simulink model "Aufgabe_5_Simu"  (Simulink 9.2)
settings: Solver=ode45  StartTime=0  StopTime=100  RelTol=1e-3  EnableMultiTasking=on
InitFcn:
  | Ts = 0.1;  % Nicht entfernen!!!
settings Model: Creator=ST  LastModifiedBy=danial
settings SolverCC: ZeroCrossAlgorithm=Adaptive
settings DataIOCC: SignalLoggingSaveFormat=Dataset
settings DebuggingCC: IgnoredZcDiagnostic=none  SolverPrmCheckMsg=warning  FcnCallInpInsideContextMsg=error
settings GRTTargetCC: CombineOutputUpdateFcns=on  GRTInterface=off
settings ConfigComp: CovSFcnEnable=off

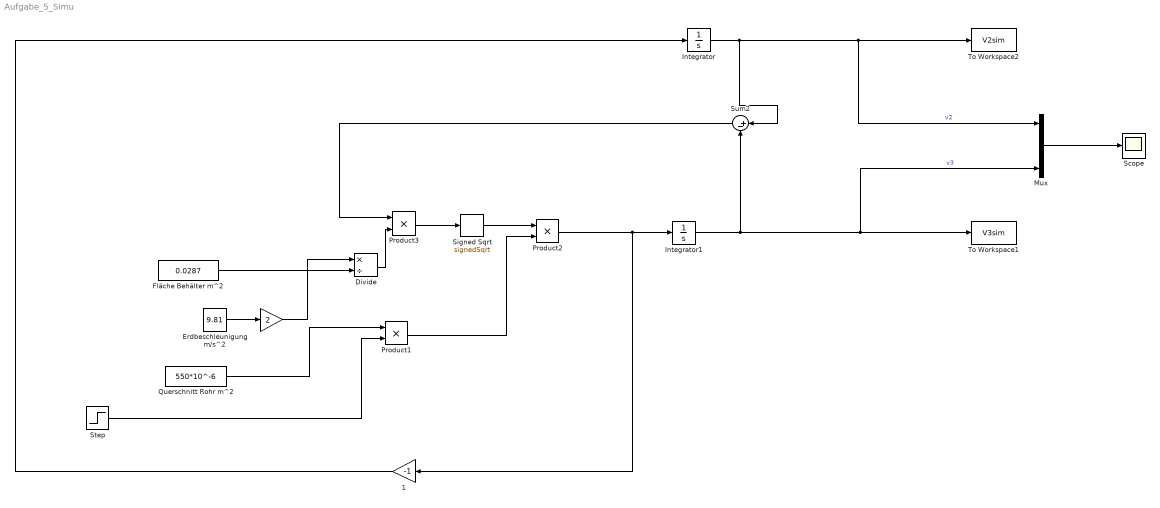
== system Aufgabe_5_Simu ==
  " " : Gain  Gain=2
  " 1" : Gain  Gain=-1
  Divide : Product  Inputs=*/
  Erdbeschleunigung m/s^2 : Constant  Value=9.81  OutDataTypeStr=double
  Fläche Behälter m^2 : Constant  Value=0.0287  OutDataTypeStr=double
  Integrator : Integrator  InitialCondition=9.2*10^-3  LimitOutput=on  UpperSaturationLimit=10*10^-3
  Integrator1 : Integrator  InitialCondition=2.6*10^-3  LimitOutput=on  UpperSaturationLimit=10*10^-3
  Mux : Mux  Inputs=3
  Product1 : Product
  Product2 : Product
  Product3 : Product
  Querschnitt Rohr m^2 : Constant  Value=550*10^-6  OutDataTypeStr=double
  Scope : Scope
  Signed Sqrt : Sqrt  Operator=signedSqrt  SaturateOnIntegerOverflow=on
  Step : Step  Time=2  SampleTime=0
  Sum2 : Sum  Inputs=|+-
  To Workspace1 : ToWorkspace  VariableName=V3sim  SampleTime=Ts
  To Workspace2 : ToWorkspace  VariableName=V2sim  SampleTime=Ts
  wires:
  Product3/1 -> Signed Sqrt/1
  Step/1 -> Product1/2
  Divide/1 -> Product3/2
  Signed Sqrt/1 -> Product2/1
  " "/1 -> Divide/1
  Product1/1 -> Product2/2
  Erdbeschleunigung m/s^2/1 -> " "/1
  Fläche Behälter m^2/1 -> Divide/2
  Querschnitt Rohr m^2/1 -> Product1/1
  Product2/1 -> " 1"/1, Integrator1/1
  Integrator/1 -> Sum2/1, Mux/1, To Workspace2/1  "v2"
  Mux/1 -> Scope/1
  Integrator1/1 -> Mux/3, To Workspace1/1, Sum2/2  "v3"
  Sum2/1 -> Product3/1
  " 1"/1 -> Integrator/1
